simulink model "sim_waypoint_test"  (R2024b)
settings: Solver=VariableStepAuto  StartTime=0.0  StopTime=inf  RelTol=1e-3
undefined symbols (not defined in the file or in its folder): Linear, mode, params, position
libraries: robotlib x3, slpidlib x3, uavalgslib x2, simulink x1, sim3dlib x1, uavsim3dlib x1, uavutilslib x1
settings Model: Creator=droneproject  LastModifiedBy=droneproject

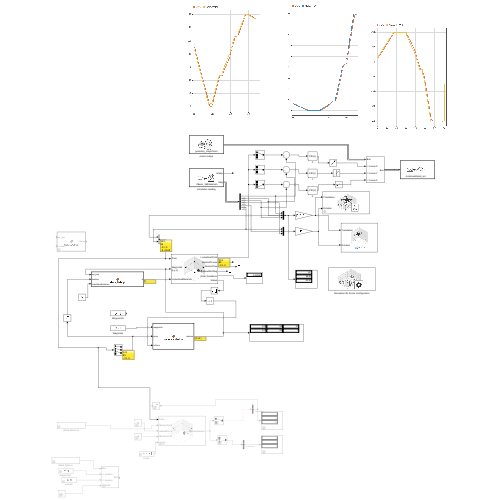
[thumbnail: Simulink's stored preview of the top-level diagram]
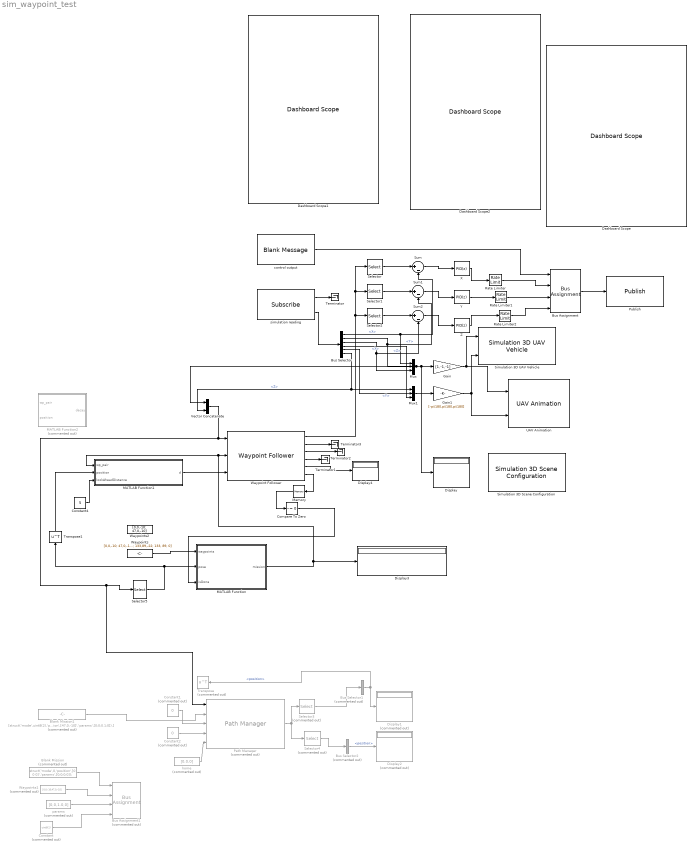
== system sim_waypoint_test ==
  Blank Mission : Constant  Commented=on  Value=struct('mode',0,'position',[0 0 0]','params',[0;0;0;0]);  OutDataTypeStr=Bus:UAVPathManagerBus
  Blank Mission1 : Constant  Commented=on  Value=[struct('mode',uint8(2),'position',[0,0,-10]','params',[0;0;0.1;0]),struct('mode',uint8(2),'position',[47,0,-10]','params',[0;0;0.1;0]),]  OutDataTypeStr=Bus:UAVPathManagerBus
  Bus Assignment : BusAssignment  AssignedSignals=Linear.X,Linear.Y,Linear.Z
  Bus Assignment1 : BusAssignment  Commented=on  AssignedSignals=position,params,mode
  Bus Selector : BusSelector  DialogController=Simulink.DDGSource_BusSelector  OutputSignals=Twist.Linear.X,Twist.Linear.Y,Twist.Linear.Z,Twist.Angular.X,Twist.Angular.Y,Twist.Angular.Z
  Bus Selector1 : BusSelector  Commented=on  OutputSignals=position
  Bus Selector2 : BusSelector  Commented=on  OutputSignals=position
  Compare To Zero : simulink/Logic and Bit Operations/Compare To Zero  relop=~=  OutDataTypeStr=boolean
  Constant : Constant  Commented=on  Value=uint8(2)
  Constant1 : Constant  Commented=on  Value=0  OutDataTypeStr=boolean
  Constant2 : Constant  Commented=on  Value=0  OutDataTypeStr=uint8
  Constant4 : Constant  Value=5
  Dashboard Scope : DashboardScope
  Dashboard Scope1 : DashboardScope
  Dashboard Scope2 : DashboardScope
  Display : Display
  Display1 : Display  Commented=on
  Display2 : Display  Commented=on
  Display3 : Display
  Display4 : Display
  Gain : Gain  Gain=[1,-1,-1]
  Gain1 : Gain  Gain=[-pi/180,pi/180,pi/180]
  MATLAB Function : MATLAB Function  TreatAsAtomicUnit=on
  MATLAB Function1 : MATLAB Function  TreatAsAtomicUnit=on
  MATLAB Function2 : MATLAB Function  Commented=on  TreatAsAtomicUnit=on
  Memory : Memory
  Mux : Mux  Inputs=3
  Mux1 : Mux  Inputs=3
  Path Manager : uavalgslib/Path Manager  Commented=on  UAVType=multirotor  LoiterRadius=25  dataType=double  inputBusName='UAVPathManagerBus'  SimulateUsing=Interpreted execution
  Publish : robotlib/Publish  topicSource=Select from ROS network  topic=/command/cmd_vel  messageType=geometry_msgs/Twist  legacyBusStruct=off  messageQueueLength=1
  Rate Limiter : RateLimiter  RisingSlewLimit=2  FallingSlewLimit=-10  SampleTimeMode=inherited
  Rate Limiter1 : RateLimiter  RisingSlewLimit=2  FallingSlewLimit=-10  SampleTimeMode=inherited
  Rate Limiter2 : RateLimiter  RisingSlewLimit=2  FallingSlewLimit=-10  SampleTimeMode=inherited
  Selector : Selector  IndexMode=Zero-based  InputPortWidth=3  IndexOptions=Index vector (dialog)  Indices=[0]  OutputSizes=1
  Selector1 : Selector  IndexMode=Zero-based  InputPortWidth=3  IndexOptions=Index vector (dialog)  Indices=[1]  OutputSizes=1
  Selector2 : Selector  IndexMode=Zero-based  InputPortWidth=3  IndexOptions=Index vector (dialog)  Indices=[2]  OutputSizes=1
  Selector3 : Selector  Commented=on  InputPortWidth=2  IndexOptions=Index vector (dialog)  Indices=[1]  OutputSizes=1
  Selector4 : Selector  Commented=on  InputPortWidth=2  IndexOptions=Index vector (dialog)  Indices=[2]  OutputSizes=1
  Selector5 : Selector  InputPortWidth=4  IndexOptions=Index vector (dialog)  Indices=[1 2 3]  OutputSizes=1
  Simulation 3D Scene Configuration : sim3dlib/Simulation 3D Scene Configuration  Priority=0  ProjectFormat=Default Scenes  SceneDesc=US city block  ProjectName=/usr/local/MATLAB/R2024b/toolbox/shared/sim3d_projects/automotive_project_linux/UE/LinuxNoEditor/VehicleSimulation.sh  ScenePath=/Game/Maps/USCityBlock  EnableOpenDRIVE=off  vehTagList={'Custom';'Scene Origin';'SimulinkVehicle1'}  vehTag=SimulinkVehicle1  FreeCameraInitialTranslation=[0, 0, 0]  FreeCameraDefaultInitialTranslation=[-6, 0, 2]  FreeCameraInitialRotation=[0, 0, 0]  FreeCameraDefaultInitialRotation=[0, -15, 0]  OpVisEn=off  Ts=1/60  EnableWindow=on  EnableRemoteAccess=off  EnableWeather=off  SunAzimuth=90  SunAltitude=40.0  EnableGeospatialSun=off  Latitude=0  Longitude=0  Date=2023-01-01  Time=10:30:00  GeoTimeZone=-5.0  SunDaylightSaving=off  wind=1  clouds=10  EnableVolumetricClouds=off  CloudCoverage=0  CloudAltitude=6  fog=0  rain=0  RaindropsEffect=off  SnowDensity=0  EnableGeospatial=off  UseTrueOrigin=off  OriginHeight=200  OriginLatitude=40.744652  OriginLongitude=-73.988864  MapStyle=Aerial  AdditionalAssetIDs=[]  UseAdvancedSunSky=off  SolarTime=11  TimeZone=-5  Day=21  Month=9  Year=2022  UseDaylightSavingTime=on  DSTStartDay=10  DSTStartMonth=3  DSTEndDay=3  DSTEndMonth=11  DSTSwitchHour=2  sensorTag=MainCamera1  sensorId=1  sensorName=MainCamera1  mountLoc=Origin  offsetFlag=off  tmountOffset=[0, 0, 0]  rmountOffset=[0, 0, 0]  HorizontalResolution=1280  VerticalResolution=720  HorizontalFOV=60  mountPoint=[0 0 0]  mountOrientation=[0 0 0]  aMode=4  ID=1  GeoTrigger=Inactive
      settings: LibrarySourceBlock=uavsim3dlib/Simulation 3D Scene Configuration
  Simulation 3D UAV Vehicle : uavsim3dlib/Simulation 3D UAV Vehicle  Priority=-1  Mesh=Quadrotor  MeshPath=/MathWorksUAVContent/UAVs/HexaRotorUAV/HexaRotor.HexaRotor  Color=Black  ActorName=SimulinkVehicle1  UseGlobalFrame=off  InitialTranslation=[0 0 0]  InitialRotation=[0 0 0]  InitialTranslationGlobal=[0 0 0]  InitialGeoOrigin=[0 0 0]  InitialRotationGlobal=[0 0 0]  SampleTime=-1  ActorType=SimulinkVehicle  ID=1  aMode=4  ActorTag=SimulinkVehicle1
  Sum : Sum  Inputs=|+-
  Sum1 : Sum  Inputs=|+-
  Sum2 : Sum  Inputs=|+-
  Terminator{,1..3} (4 alike) : Terminator
  Transpose : Math  Commented=on  Operator=transpose
  Transpose1 : Math  Operator=transpose
  UAV Animation : uavutilslib/UAV Animation  NumUAV=1  DynamicUAVConfig=off  UAVType=Multirotor  UAVSize=1  UAVColor=[1 0 0]  UAVTrajectoryAlpha=1  InertialZDirection=Up  RotationFormat=Euler ZYX  DrawMarkers=off  SampleTime=-1
  Vector Concatenate : Concatenate
  Waypoint Follower : uavalgslib/Waypoint Follower  UAVType=multirotor  StartFrom=first  TransitionRadiusSource=internal  TransitionRadius=0.03  MinLookaheadDistance=0.1  HoverAtLastWaypoint=on  YawInput=off  ShowCrossTrackErrorOutput=on  ShowStatusOutput=on  SimulateUsing=Interpreted execution
  Waypoints : Constant  Value=[0,0,-10; 47,0,-10; 107,9,-15; 140,43,-22; 133,89,-22; 133, 89, 0]  VectorParams1D=off
  Waypoints1 : Constant  Commented=on  Value=[0,0,-10;47,0,-10]
  Waypoints2 : Constant  Value=[0,0,-10; 47,0,-10]  VectorParams1D=off
  X : slpidlib/PID Controller  Controller=PID  Form=Parallel  TimeDomain=Discrete-time  UseExternalTs=off  SampleTime=0.01  IntegratorMethod=Forward Euler  FilterMethod=Forward Euler  ControllerParametersSource=internal  P=0.7  I=0  UseKiTs=off  D=0.08  UseExternalDerivativeSource=off  N=3  UseFilter=on  TunerSelectOption=Frequency Response Based  InitialConditionSource=internal  InitialConditionForIntegrator=0  InitialConditionForFilter=0  DifferentiatorICPrevScaledInput=0  ExternalReset=none  TrackingMode=off  Kt=1  LimitOutput=off  SatLimitsSource=internal  UpperSaturationLimit=1  LowerSaturationLimit=-1  LinearizeAsGain=on  AntiWindupMode=none  Kb=1  LimitIntegrator=off  UpperIntegratorSaturationLimit=inf  LowerIntegratorSaturationLimit=-inf  POutMin=[]  POutMax=[]  IOutMin=[]  IOutMax=[]  DOutMin=[]  DOutMax=[]  NOutMin=[]  NOutMax=[]  SumOutMin=[]  SumOutMax=[]  SaturationOutMin=[]  SaturationOutMax=[]  PParamMin=[]  PParamMax=[]  IParamMin=[]  IParamMax=[]  DParamMin=[]  DParamMax=[]  NParamMin=[]  NParamMax=[]  KbParamMin=[]  KbParamMax=[]  KtParamMin=[]  KtParamMax=[]  KbOutMin=[]  KbOutMax=[]  KtOutMin=[]  KtOutMax=[]  IntegratorOutMin=[]  IntegratorOutMax=[]  FilterOutMin=[]  FilterOutMax=[]  SumI1OutMin=[]  SumI1OutMax=[]  SumI2OutMin=[]  SumI2OutMax=[]  SumI3OutMin=[]  SumI3OutMax=[]  SumI4OutMin=[]  SumI4OutMax=[]  SumDOutMin=[]  SumDOutMax=[]  DifferentiatorOutMin=[]  DifferentiatorOutMax=[]  FilterDiffOutCoefMin=[]  FilterDiffOutCoefMax=[]  ReciprocalOutMin=[]  ReciprocalOutMax=[]  SumDenOutMin=[]  SumDenOutMax=[]  SumNumOutMin=[]  SumNumOutMax=[]  DivideOutMin=[]  DivideOutMax=[]  UdiffTsProdOutMin=[]  UdiffTsProdOutMax=[]  NTsProdOutMin=[]  NTsProdOutMax=[]  UintegralTsProdOutMin=[]  UintegralTsProdOutMax=[]  UngainTsProdOutMin=[]  UngainTsProdOutMax=[]  ClampingZeroOutDataTypeStr=Inherit: Inherit via back propagation  ClampingZeroOutMin=[]  ClampingZeroOutMax=[]  FilterDenConstantOutDataTypeStr=Inherit: Inherit via back propagation  FilterDenConstantOutMin=[]  FilterDenConstantOutMax=[]  PCopyOutDataTypeStr=Inherit: Inherit via back propagation  PCopyOutMin=[]  PCopyOutMax=[]  NCopyOutDataTypeStr=Inherit: Inherit via back propagation  NCopyOutMin=[]  NCopyOutMax=[]  IntegratorContinuousStateAttributes=''  IntegratorStateMustResolveToSignalObject=off  IntegratorRTWStateStorageClass=Auto  FilterContinuousStateAttributes=''  FilterStateMustResolveToSignalObject=off  FilterRTWStateStorageClass=Auto  ParallelPVariant=InternalParameters  IdealPVariant=Disabled  IVariant=InternalParameters  DVariant=InternalParameters  IntegratorVariant=Discrete  SatVariant=Disabled  AWVariant=Passthrough  PCopyVariant=Disabled  TRVariant=Disabled  FdbkBlocksVariant=Forward  IdealPFdbkVariant=Disabled  SatFdbkVariant=Disabled  DerivativeFilterVariant=ForwardEulerFilter  NVariant=InternalParameters  NCopyVariant=Disabled  FilterICVariant=InternalICsFilter  IntegratorICVariant=InternalICs  ExternalResetVariant=Disabled  TRSumVariant=Passthrough  SumFdbkVariant=Disabled  SumVariant=Sum_PID  TsampFilterVariant=InternalTs  TsampNgainVariant=Passthrough  TsampIntegralVariant=Disabled_SignalSpec  ExternalSaturationOutDataTypeStr=Inherit: Same as second input  DerivativeSourceVariant=ErrorSignal  PreIntVariant=InternalPreInt
  Y : slpidlib/PID Controller  Controller=PID  Form=Parallel  TimeDomain=Discrete-time  UseExternalTs=off  SampleTime=0.01  IntegratorMethod=Forward Euler  FilterMethod=Forward Euler  ControllerParametersSource=internal  P=0.7  I=0  UseKiTs=off  D=0.08  UseExternalDerivativeSource=off  N=3  UseFilter=on  TunerSelectOption=Frequency Response Based  InitialConditionSource=internal  InitialConditionForIntegrator=0  InitialConditionForFilter=0  DifferentiatorICPrevScaledInput=0  ExternalReset=none  TrackingMode=off  Kt=1  LimitOutput=off  SatLimitsSource=internal  UpperSaturationLimit=1  LowerSaturationLimit=-1  LinearizeAsGain=on  AntiWindupMode=none  Kb=1  LimitIntegrator=off  UpperIntegratorSaturationLimit=inf  LowerIntegratorSaturationLimit=-inf  POutMin=[]  POutMax=[]  IOutMin=[]  IOutMax=[]  DOutMin=[]  DOutMax=[]  NOutMin=[]  NOutMax=[]  SumOutMin=[]  SumOutMax=[]  SaturationOutMin=[]  SaturationOutMax=[]  PParamMin=[]  PParamMax=[]  IParamMin=[]  IParamMax=[]  DParamMin=[]  DParamMax=[]  NParamMin=[]  NParamMax=[]  KbParamMin=[]  KbParamMax=[]  KtParamMin=[]  KtParamMax=[]  KbOutMin=[]  KbOutMax=[]  KtOutMin=[]  KtOutMax=[]  IntegratorOutMin=[]  IntegratorOutMax=[]  FilterOutMin=[]  FilterOutMax=[]  SumI1OutMin=[]  SumI1OutMax=[]  SumI2OutMin=[]  SumI2OutMax=[]  SumI3OutMin=[]  SumI3OutMax=[]  SumI4OutMin=[]  SumI4OutMax=[]  SumDOutMin=[]  SumDOutMax=[]  DifferentiatorOutMin=[]  DifferentiatorOutMax=[]  FilterDiffOutCoefMin=[]  FilterDiffOutCoefMax=[]  ReciprocalOutMin=[]  ReciprocalOutMax=[]  SumDenOutMin=[]  SumDenOutMax=[]  SumNumOutMin=[]  SumNumOutMax=[]  DivideOutMin=[]  DivideOutMax=[]  UdiffTsProdOutMin=[]  UdiffTsProdOutMax=[]  NTsProdOutMin=[]  NTsProdOutMax=[]  UintegralTsProdOutMin=[]  UintegralTsProdOutMax=[]  UngainTsProdOutMin=[]  UngainTsProdOutMax=[]  ClampingZeroOutDataTypeStr=Inherit: Inherit via back propagation  ClampingZeroOutMin=[]  ClampingZeroOutMax=[]  FilterDenConstantOutDataTypeStr=Inherit: Inherit via back propagation  FilterDenConstantOutMin=[]  FilterDenConstantOutMax=[]  PCopyOutDataTypeStr=Inherit: Inherit via back propagation  PCopyOutMin=[]  PCopyOutMax=[]  NCopyOutDataTypeStr=Inherit: Inherit via back propagation  NCopyOutMin=[]  NCopyOutMax=[]  IntegratorContinuousStateAttributes=''  IntegratorStateMustResolveToSignalObject=off  IntegratorRTWStateStorageClass=Auto  FilterContinuousStateAttributes=''  FilterStateMustResolveToSignalObject=off  FilterRTWStateStorageClass=Auto  ParallelPVariant=InternalParameters  IdealPVariant=Disabled  IVariant=InternalParameters  DVariant=InternalParameters  IntegratorVariant=Discrete  SatVariant=Disabled  AWVariant=Passthrough  PCopyVariant=Disabled  TRVariant=Disabled  FdbkBlocksVariant=Forward  IdealPFdbkVariant=Disabled  SatFdbkVariant=Disabled  DerivativeFilterVariant=ForwardEulerFilter  NVariant=InternalParameters  NCopyVariant=Disabled  FilterICVariant=InternalICsFilter  IntegratorICVariant=InternalICs  ExternalResetVariant=Disabled  TRSumVariant=Passthrough  SumFdbkVariant=Disabled  SumVariant=Sum_PID  TsampFilterVariant=InternalTs  TsampNgainVariant=Passthrough  TsampIntegralVariant=Disabled_SignalSpec  ExternalSaturationOutDataTypeStr=Inherit: Same as second input  DerivativeSourceVariant=ErrorSignal  PreIntVariant=InternalPreInt
  Z : slpidlib/PID Controller  Controller=PID  Form=Parallel  TimeDomain=Discrete-time  UseExternalTs=off  SampleTime=0.01  IntegratorMethod=Forward Euler  FilterMethod=Forward Euler  ControllerParametersSource=internal  P=0.7  I=0  UseKiTs=off  D=0.08  UseExternalDerivativeSource=off  N=3  UseFilter=on  TunerSelectOption=Frequency Response Based  InitialConditionSource=internal  InitialConditionForIntegrator=0  InitialConditionForFilter=0  DifferentiatorICPrevScaledInput=0  ExternalReset=none  TrackingMode=off  Kt=1  LimitOutput=off  SatLimitsSource=internal  UpperSaturationLimit=1  LowerSaturationLimit=-1  LinearizeAsGain=on  AntiWindupMode=none  Kb=1  LimitIntegrator=off  UpperIntegratorSaturationLimit=inf  LowerIntegratorSaturationLimit=-inf  POutMin=[]  POutMax=[]  IOutMin=[]  IOutMax=[]  DOutMin=[]  DOutMax=[]  NOutMin=[]  NOutMax=[]  SumOutMin=[]  SumOutMax=[]  SaturationOutMin=[]  SaturationOutMax=[]  PParamMin=[]  PParamMax=[]  IParamMin=[]  IParamMax=[]  DParamMin=[]  DParamMax=[]  NParamMin=[]  NParamMax=[]  KbParamMin=[]  KbParamMax=[]  KtParamMin=[]  KtParamMax=[]  KbOutMin=[]  KbOutMax=[]  KtOutMin=[]  KtOutMax=[]  IntegratorOutMin=[]  IntegratorOutMax=[]  FilterOutMin=[]  FilterOutMax=[]  SumI1OutMin=[]  SumI1OutMax=[]  SumI2OutMin=[]  SumI2OutMax=[]  SumI3OutMin=[]  SumI3OutMax=[]  SumI4OutMin=[]  SumI4OutMax=[]  SumDOutMin=[]  SumDOutMax=[]  DifferentiatorOutMin=[]  DifferentiatorOutMax=[]  FilterDiffOutCoefMin=[]  FilterDiffOutCoefMax=[]  ReciprocalOutMin=[]  ReciprocalOutMax=[]  SumDenOutMin=[]  SumDenOutMax=[]  SumNumOutMin=[]  SumNumOutMax=[]  DivideOutMin=[]  DivideOutMax=[]  UdiffTsProdOutMin=[]  UdiffTsProdOutMax=[]  NTsProdOutMin=[]  NTsProdOutMax=[]  UintegralTsProdOutMin=[]  UintegralTsProdOutMax=[]  UngainTsProdOutMin=[]  UngainTsProdOutMax=[]  ClampingZeroOutDataTypeStr=Inherit: Inherit via back propagation  ClampingZeroOutMin=[]  ClampingZeroOutMax=[]  FilterDenConstantOutDataTypeStr=Inherit: Inherit via back propagation  FilterDenConstantOutMin=[]  FilterDenConstantOutMax=[]  PCopyOutDataTypeStr=Inherit: Inherit via back propagation  PCopyOutMin=[]  PCopyOutMax=[]  NCopyOutDataTypeStr=Inherit: Inherit via back propagation  NCopyOutMin=[]  NCopyOutMax=[]  IntegratorContinuousStateAttributes=''  IntegratorStateMustResolveToSignalObject=off  IntegratorRTWStateStorageClass=Auto  FilterContinuousStateAttributes=''  FilterStateMustResolveToSignalObject=off  FilterRTWStateStorageClass=Auto  ParallelPVariant=InternalParameters  IdealPVariant=Disabled  IVariant=InternalParameters  DVariant=InternalParameters  IntegratorVariant=Discrete  SatVariant=Disabled  AWVariant=Passthrough  PCopyVariant=Disabled  TRVariant=Disabled  FdbkBlocksVariant=Forward  IdealPFdbkVariant=Disabled  SatFdbkVariant=Disabled  DerivativeFilterVariant=ForwardEulerFilter  NVariant=InternalParameters  NCopyVariant=Disabled  FilterICVariant=InternalICsFilter  IntegratorICVariant=InternalICs  ExternalResetVariant=Disabled  TRSumVariant=Passthrough  SumFdbkVariant=Disabled  SumVariant=Sum_PID  TsampFilterVariant=InternalTs  TsampNgainVariant=Passthrough  TsampIntegralVariant=Disabled_SignalSpec  ExternalSaturationOutDataTypeStr=Inherit: Same as second input  DerivativeSourceVariant=ErrorSignal  PreIntVariant=InternalPreInt
  control output : robotlib/Blank Message  messageClass=Message  entityType=geometry_msgs/Twist  messageType=geometry_msgs/Twist  SampleTime=inf  legacyBusStruct=off
  home : Constant  Commented=on  Value=[0,0,0]
  params : Constant  Commented=on  Value=[0,0,1.0,0]
  simulation reading : robotlib/Subscribe  topicSource=Select from ROS network  topic=/Mavic_3M/state/sim  messageType=geometry_msgs/TwistStamped  SampleTime=-1  legacyBusStruct=off  messageQueueLength=1
  wires:
  simulation reading/2 -> Bus Selector/1
  simulation reading/1 -> Terminator/1
  control output/1 -> Bus Assignment/1
  Bus Assignment/1 -> Publish/1
  Sum/1 -> X/1
  Sum1/1 -> Y/1
  Sum2/1 -> Z/1
  Bus Selector/1 -> Mux/1, Sum/2  "<X>"
  Bus Selector/2 -> Mux/2, Sum1/2  "<Y>"
  Bus Selector/3 -> Sum2/2, Mux/3  "<Z>"
  Mux1/1 -> Gain1/1
  Gain/1 -> UAV Animation/1, Simulation 3D UAV Vehicle/1
  Gain1/1 -> UAV Animation/2, Simulation 3D UAV Vehicle/2
  Bus Selector/5 -> Mux1/2  "<Y>"
  Bus Selector/4 -> Mux1/3  "<X>"
  Bus Selector/6 -> Mux1/1, Vector Concatenate/2  "<Z>"
  Vector Concatenate/1 -> Selector5/1, Path Manager/1, Waypoint Follower/1
  Waypoint Follower/3 -> Terminator2/1
  Waypoint Follower/2 -> Terminator3/1
  Waypoint Follower/1 -> Selector1/1, Selector/1, Selector2/1
  Mux/1 -> Gain/1, Display/1, Vector Concatenate/1
  Blank Mission/1 -> Bus Assignment1/1
  Constant/1 -> Bus Assignment1/4
  Waypoints1/1 -> Bus Assignment1/2
  params/1 -> Bus Assignment1/3
  Path Manager/1 -> Selector4/1, Selector3/1
  Selector4/1 -> Bus Selector2/1
  Selector3/1 -> Bus Selector1/1
  Bus Selector1/1 -> Transpose/1, Display1/1  "<position>"
  Bus Selector2/1 -> Display2/1  "<position>"
  home/1 -> Path Manager/5
  Constant1/1 -> Path Manager/3
  Constant2/1 -> Path Manager/4
  Blank Mission1/1 -> Path Manager/2
  MATLAB Function/1(mission) -> Waypoint Follower/2, MATLAB Function1/1(wp_pair), Display3/1
  Compare To Zero/1 -> MATLAB Function/3(isDone)
  Selector5/1 -> MATLAB Function/2(pose), Transpose1/1
  Selector1/1 -> Sum1/1
  Selector2/1 -> Sum2/1
  Selector/1 -> Sum/1
  Transpose1/1 -> MATLAB Function1/2(position)
  Waypoint Follower/6 -> Memory/1
  Waypoint Follower/5 -> Display4/1
  Waypoints/1 -> MATLAB Function/1(waypoints)
  Constant4/1 -> MATLAB Function1/3(lookAheadDistance)
  X/1 -> Rate Limiter/1
  Y/1 -> Rate Limiter1/1
  Z/1 -> Rate Limiter2/1
  Waypoint Follower/4 -> Terminator1/1
  Rate Limiter/1 -> Bus Assignment/2
  Rate Limiter1/1 -> Bus Assignment/3
  Rate Limiter2/1 -> Bus Assignment/4
  Memory/1 -> Compare To Zero/1
  MATLAB Function1/1(d) -> Waypoint Follower/3

== matlab function sim_waypoint_test/MATLAB Function1 ==
  data: wp_pair input; d output; position input; lookAheadDistance input
function d = decayDebug(wp_pair, position, lookAheadDistance)
%#codegen
prevWP = wp_pair(1,:);
nextWP = wp_pair(2,:);

distToStart = norm(position - prevWP);
distToEnd   = norm(position - nextWP);

%thresh = 5;
if distToStart >= distToEnd
    x = distToEnd;
    if x <= lookAheadDistance
        d = x+0.2;
    else
        d = lookAheadDistance;
    end
else
    %x = distToStart;
    d = lookAheadDistance;
end






%if x <= thresh
%    decay = x*(2*thresh-x)/thresh^2;
%else
%  decay = 1;
%end



end

== matlab function sim_waypoint_test/MATLAB Function ==
  data: waypoints input; mission output; pose input; isDone input
% MATLAB Function Block: generateMission
% Inputs:
%   waypoints   - Nx3 matrix of [x y z] waypoints
%   pose        - 1x3 current [x y z] position
%   isDone      - scalar (0 or 1), indicates waypoint reached
% Output:
%   mission     - 2x3 matrix: [previous_wp; target_wp]

function mission = generateMission(waypoints, pose, isDone)
%#codegen
% Preallocate output for codegen
mission = zeros(2,3,'like',waypoints);

persistent idx prevWP prevDone nWPs

% Initialize or reset on waypoint count change
if isempty(nWPs)
    nWPs = size(waypoints,1);
end
if isempty(idx) || nWPs ~= size(waypoints,1)
    idx      = 1;
    prevWP   = pose;       % start from initial pose
    prevDone = false;
    nWPs     = size(waypoints,1);
end

% Detect rising edge of isDone
if isDone && ~prevDone
    wait
    % Advance previous to current target
    prevWP = waypoints(idx, :);
    % Increment index, cap at end
    idx = min(idx + 1, nWPs);
end
% Store current isDone state
prevDone = isDone;

% Output previous and current target waypoints
mission(1, :) = prevWP;
mission(2, :) = waypoints(idx, :);
end

== matlab function sim_waypoint_test/MATLAB Function2 ==
  data: wp_pair input; decay output; position input
function decay = decayDebug(wp_pair, position)
%#codegen
prevWP = wp_pair(1,:);
nextWP = wp_pair(2,:);

distToStart = norm(position - prevWP);
distToEnd   = norm(position - nextWP);

thresh = 5;
if distToStart >= distToEnd
    x = distToEnd;
else
    x = distToStart;
end


if x <= thresh
    decay = x*(2*thresh-x)/thresh^2;
else
  decay = 1;
end



end
